simulink model "ayazTethers_th"  (R2018b)
settings: Solver=VariableStepAuto  StartTime=0.0  StopTime=0  RelTol=1e-3
values from neighbouring files (symbols this model uses):
  bdyAngAccel = [0 0 0]'    [ayazTethers_ts.m]
  bdyAngVel = [0 0 0]'    [ayazTethers_ts.m]
  eulAng = [0 0 0]'    [ayazTethers_ts.m]
  liftBdyAccel = [0 0 0]'    [ayazTethers_ts.m]
  platformAng = 0    [ayazTethers_ts.m]
  platformAngAccel = 0    [ayazTethers_ts.m]
  platformAngVel = 0    [ayazTethers_ts.m]
libraries: ayazTethers_cl x1
settings Model: Creator=mcobb  LastModifiedBy=mcobb

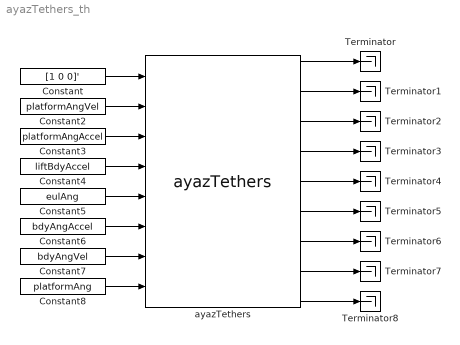
== system ayazTethers_th ==
  Constant : Constant  Value=[1 0 0]'
  Constant2 : Constant  Value=platformAngVel
  Constant3 : Constant  Value=platformAngAccel
  Constant4 : Constant  Value=liftBdyAccel
  Constant5 : Constant  Value=eulAng
  Constant6 : Constant  Value=bdyAngAccel
  Constant7 : Constant  Value=bdyAngVel
  Constant8 : Constant  Value=platformAng
  Terminator{,1..8} (9 alike) : Terminator
  ayazTethers : ayazTethers_cl/ayazTethers  SystemSampleTime=-1
  wires:
  Constant/1 -> ayazTethers/1
  ayazTethers/1 -> Terminator/1
  ayazTethers/4 -> Terminator3/1
  ayazTethers/3 -> Terminator2/1
  ayazTethers/2 -> Terminator1/1
  ayazTethers/6 -> Terminator5/1
  ayazTethers/5 -> Terminator4/1
  ayazTethers/7 -> Terminator6/1
  ayazTethers/8 -> Terminator7/1
  ayazTethers/9 -> Terminator8/1
  Constant2/1 -> ayazTethers/2
  Constant3/1 -> ayazTethers/3
  Constant4/1 -> ayazTethers/4
  Constant5/1 -> ayazTethers/5
  Constant6/1 -> ayazTethers/6
  Constant7/1 -> ayazTethers/7
  Constant8/1 -> ayazTethers/8
